simulink model "ex_anti_windup_PI"  (R2019b)
settings: Solver=VariableStepAuto  StartTime=0.0  StopTime=60  RelTol=1e-3  EnableMultiTasking=on
StopFcn:
  | figure(1);
  | 
  | subplot(211);
  | plot(r.time,r.data,y1.time,y1.data,'LineWidth',1);
  | title('Sans dispositif anti-windup');
  | ylabel('r(t) , y(t)');
  | xlabel('Temps (s)');
  | 
  | subplot(212);
  | plot(uc1.time,uc1.data,u1.time,u1.data,'LineWidth',1);
  | ylabel('u_c(t) , u(t)');
  | xlabel('Temps (s)');
  | 
  | figure(2);
  | 
  | subplot(211);
  | plot(r.time,r.data,y2.time,y2.data,'LineWidth',1);
  | title('Avec dispositif anti-windup');
  | ylabel('r(t) , y(t)');
  | xlabel('Temps (s)');
  | 
  | subplot(212);
  | plot(uc2.time,uc2.data,u2.time,u2.data,'LineWidth',1);
  | ylabel('u_c(t) , u(t)');
  | xlabel('Temps (s)');
settings Model: Creator=epoulin  LastModifiedBy=eric
settings DataIOCC: LimitDataPoints=on  SaveFormat=Array  SignalLoggingSaveFormat=ModelDataLogs  SaveTime=off  ReturnWorkspaceOutputs=off
settings OptimizationCC: BooleanDataType=off  ExpressionDepthLimit=2147483647  InitFltsAndDblsToZero=on  LifeSpan=inf
settings DebuggingCC: SaveWithParameterizedLinksMsg=none  UnderspecifiedInitializationDetection=Classic  MergeDetectMultiDrivingBlocksExec=none  SignalResolutionControl=TryResolveAllWithWarning  MultiTaskDSMMsg=warning  MultiTaskCondExecSysMsg=none  FcnCallInpInsideContextMsg=warning  StateNameClashWarn=warning  SFUnexpectedBacktrackingDiag=warning  SFNoUnconditionalDefaultTransitionDiag=warning  SFExecutionAtInitializationDiag=none  ArithmeticOperatorsInVariantConditions=warning
settings HardwareCC: ProdBitPerPointer=32  ProdBitPerSizeT=32  ProdBitPerPtrDiffT=32  ProdLargestAtomicFloat=None  ProdIntDivRoundTo=Undefined  ProdEndianess=Unspecified  ProdWordSize=32  ProdHWDeviceType=32-bit Generic  TargetUnknown=on
settings ModelReferenceCC: PropagateSignalLabelsOutOfModel=off
settings SFSimCC: SimUseLocalCustomCode=off  CustomCodeUndefinedFunction=UseInterfaceOnly
settings RTWCC: RTWUseLocalCustomCode=off
settings CodeAppCC: StateflowObjectComments=on
settings GRTTargetCC: TargetFcnLib=ansi_tfl_tmw.mat  TargetLangStandard=C89/C90 (ANSI)  ModelReferenceCompliant=off  GeneratePreprocessorConditionals=Disable all  CombineOutputUpdateFcns=off  MatFileLogging=off  GRTInterface=on
settings ConfigComp: CovMetricSettings=dw  CovHtmlReporting=on  CovSaveCumulativeToWorkspaceVar=on  CovSaveSingleToWorkspaceVar=on  CovExternalEMLEnable=off  CovSFcnEnable=off

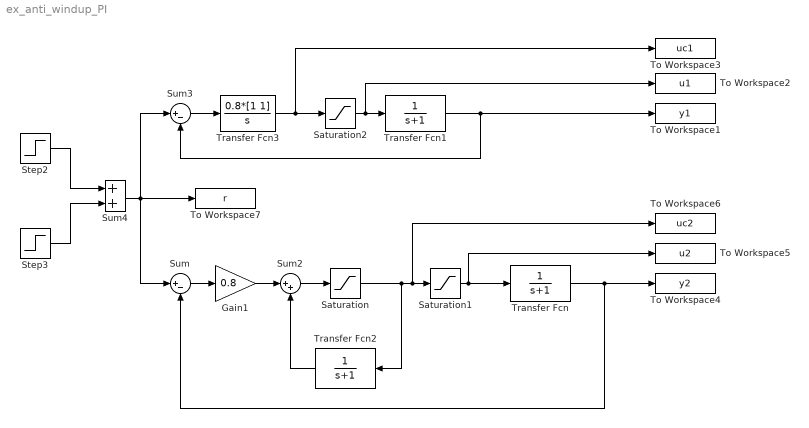
== system ex_anti_windup_PI ==
  Gain1 : Gain  Gain=0.8  SaturateOnIntegerOverflow=on  OutDataTypeStr=Inherit: Same as input  ParamDataTypeStr=Inherit: Same as input
  Saturation : Saturate
  Saturation1 : Saturate
  Saturation2 : Saturate
  Step2 : Step  SampleTime=0
  Step3 : Step  Time=15  After=-0.75  SampleTime=0
  Sum : Sum  Inputs=|+-  SaturateOnIntegerOverflow=on  InputSameDT=on  OutDataTypeStr=Inherit: Same as first input
  Sum2 : Sum  Inputs=|++  SaturateOnIntegerOverflow=on  InputSameDT=on  OutDataTypeStr=Inherit: Same as first input
  Sum3 : Sum  Inputs=|+-  SaturateOnIntegerOverflow=on  InputSameDT=on  OutDataTypeStr=Inherit: Same as first input
  Sum4 : Sum  SaturateOnIntegerOverflow=on  InputSameDT=on  OutDataTypeStr=Inherit: Same as first input
  To Workspace1 : ToWorkspace  VariableName=y1  SaveFormat=Timeseries  SampleTime=-1
  To Workspace2 : ToWorkspace  VariableName=u1  SaveFormat=Timeseries  SampleTime=-1
  To Workspace3 : ToWorkspace  VariableName=uc1  SaveFormat=Timeseries  SampleTime=-1
  To Workspace4 : ToWorkspace  VariableName=y2  SaveFormat=Timeseries  SampleTime=-1
  To Workspace5 : ToWorkspace  VariableName=u2  SaveFormat=Timeseries  SampleTime=-1
  To Workspace6 : ToWorkspace  VariableName=uc2  SaveFormat=Timeseries  SampleTime=-1
  To Workspace7 : ToWorkspace  VariableName=r  SaveFormat=Timeseries  SampleTime=-1
  Transfer Fcn : TransferFcn  Denominator=[1 1]
  Transfer Fcn1 : TransferFcn  Denominator=[1 1]
  Transfer Fcn2 : TransferFcn  Numerator=1  Denominator=[1 1]
  Transfer Fcn3 : TransferFcn  Numerator=0.8*[1 1]  Denominator=[1 0]
  wires:
  Saturation/1 -> Transfer Fcn2/1, Saturation1/1, To Workspace6/1
  Transfer Fcn/1 -> Sum/2, To Workspace4/1
  Transfer Fcn2/1 -> Sum2/2
  Saturation1/1 -> Transfer Fcn/1, To Workspace5/1
  Sum3/1 -> Transfer Fcn3/1
  Transfer Fcn3/1 -> Saturation2/1, To Workspace3/1
  Saturation2/1 -> Transfer Fcn1/1, To Workspace2/1
  Transfer Fcn1/1 -> Sum3/2, To Workspace1/1
  Step2/1 -> Sum4/1
  Step3/1 -> Sum4/2
  Sum4/1 -> Sum3/1, Sum/1, To Workspace7/1
  Sum2/1 -> Saturation/1
  Gain1/1 -> Sum2/1
  Sum/1 -> Gain1/1
